simulink model "chap05"  (R2021a)
settings: Solver=FixedStepDiscrete  StartTime=0.0  StopTime=inf  FixedStep=0.001  RelTol=1e-3
undefined symbols (not defined in the file): DiscIntNeverNeededParam, Header, Pose, X, Y, Z
libraries: robotlib x31
(part 9 of 9)

== matlab function chap05/Subsystem16/Subsystem3/Subsystem9/Subsystem/MATLAB Function ==
  data: u1 input; y output; u2 input
function y = fcn(u1,u2)


if (u1==u2)
    y = 0;
else
    y = 1;
end

== matlab function chap05/Subsystem16/Subsystem3/Subsystem3/MATLAB Function ==
  data: u input; y output
function y = fcn(u)

y = u;

if y==0
    y=10e-15;
end

== matlab function chap05/Subsystem16/Subsystem3/Subsystem3/MATLAB Function1 ==
  data: u input; y output
function y = fcn(u)

y = u;

if y==0
    y=10e-15;
end

== matlab function chap05/Subsystem16/Subsystem3/Subsystem3/MATLAB Function2 ==
  data: u input; y output
function y = fcn(u)

y = u;

if y==0
    y=10e-15;
end

== matlab function chap05/Subsystem16/Subsystem3/Subsystem3/Subsystem/MATLAB Function ==
  data: u input; y output
function y = fcn(u)

y = norm(u);

== matlab function chap05/Subsystem16/Subsystem3/Subsystem8/MATLAB Function1 ==
  data: u input; y output
function y = fcn(u)

y = norm(u);

== matlab function chap05/Subsystem16/Subsystem3/Subsystem3/Subsystem1/MATLAB Function ==
  data: u input; y output
function y = fcn(u)

y = norm(u)^(1/2);

== matlab function chap05/Subsystem16/Subsystem5/Subsystem11/Subsystem/MATLAB Function ==
  data: u1 input; y output; u2 input
function y = fcn(u1,u2)


if (u1==u2)
    y = 0;
else
    y = 1;
end

== matlab function chap05/Subsystem16/Subsystem5/Subsystem3/MATLAB Function ==
  data: u input; y output
function y = fcn(u)

y = u;

if y==0
    y=10e-15;
end

== matlab function chap05/Subsystem16/Subsystem5/Subsystem3/MATLAB Function1 ==
  data: u input; y output
function y = fcn(u)

y = u;

if y==0
    y=10e-15;
end

== matlab function chap05/Subsystem16/Subsystem5/Subsystem10/MATLAB Function ==
  data: u input; utk input; nrom output
function nrom = fcn(u,utk)

e = utk-u;
nrom = norm(e);

== matlab function chap05/Subsystem16/Subsystem5/Subsystem3/MATLAB Function2 ==
  data: u input; y output
function y = fcn(u)

y = u;

if y==0
    y=10e-15;
end

== matlab function chap05/Subsystem16/Subsystem5/Subsystem3/Subsystem/MATLAB Function ==
  data: u input; y output
function y = fcn(u)

y = norm(u);

== matlab function chap05/Subsystem16/Subsystem5/Subsystem3/Subsystem1/MATLAB Function ==
  data: u input; y output
function y = fcn(u)

y = norm(u)^(1/2);

== matlab function chap05/Subsystem16/Subsystem5/Subsystem4/Subsystem/MATLAB Function ==
  data: u1 input; y output; u2 input
function y = fcn(u1,u2)


if (u1==u2)
    y = 0;
else
    y = 1;
end

== matlab function chap05/Subsystem16/Subsystem5/Subsystem9/Subsystem/MATLAB Function ==
  data: u1 input; y output; u2 input
function y = fcn(u1,u2)


if (u1==u2)
    y = 0;
else
    y = 1;
end

== matlab function chap05/Subsystem16/Subsystem5/Subsystem7/MATLAB Function ==
  data: u input; y output
function y = fcn(u)

y = norm(u);

== matlab function chap05/Subsystem16/Subsystem6/Subsystem4/Subsystem/MATLAB Function ==
  data: u1 input; y output; u2 input
function y = fcn(u1,u2)


if (u1==u2)
    y = 0;
else
    y = 1;
end

== matlab function chap05/Subsystem16/Subsystem6/Subsystem5/Subsystem/MATLAB Function ==
  data: u1 input; y output; u2 input
function y = fcn(u1,u2)


if (u1==u2)
    y = 0;
else
    y = 1;
end

== matlab function chap05/Subsystem16/Subsystem6/Subsystem7/Subsystem/MATLAB Function ==
  data: u1 input; y output; u2 input
function y = fcn(u1,u2)


if (u1==u2)
    y = 0;
else
    y = 1;
end

== matlab function chap05/Subsystem16/Subsystem1/Subsystem11/Subsystem/MATLAB Function ==
  data: u1 input; y output; u2 input
function y = fcn(u1,u2)


if (u1==u2)
    y = 0;
else
    y = 1;
end

== matlab function chap05/Subsystem16/Subsystem1/Subsystem5/Subsystem/MATLAB Function ==
  data: u1 input; y output; u2 input
function y = fcn(u1,u2)


if (u1==u2)
    y = 0;
else
    y = 1;
end

== matlab function chap05/Subsystem16/Subsystem1/Subsystem9/Subsystem/MATLAB Function ==
  data: u1 input; y output; u2 input
function y = fcn(u1,u2)


if (u1==u2)
    y = 0;
else
    y = 1;
end

== matlab function chap05/Subsystem16/Subsystem12/MATLAB Function ==
  data: u input; y output
function y = fcn(u)

y = norm(u);

== matlab function chap05/Subsystem16/Subsystem12/MATLAB Function2 ==
  data: u input; y output
function y = fcn(u)

y = norm(u);

== matlab function chap05/Subsystem16/Subsystem12/MATLAB Function3 ==
  data: u input; y output
function y = fcn(u)

y = norm(u);

== matlab function chap05/Subsystem16/Subsystem5/Subsystem7/MATLAB Function1 ==
  data: u input; y output
function y = fcn(u)

y = norm(u);

== matlab function chap05/Subsystem16/Subsystem14/MATLAB Function ==
  data: u input; y output
function y = fcn(u)

y = norm(u);

== matlab function chap05/Subsystem16/Subsystem14/MATLAB Function2 ==
  data: u input; y output
function y = fcn(u)

y = norm(u);

== matlab function chap05/Subsystem16/Subsystem14/MATLAB Function3 ==
  data: u input; y output
function y = fcn(u)

y = norm(u);

== matlab function chap05/Subsystem16/Subsystem15/MATLAB Function ==
  data: u input; y output
function y = fcn(u)

y = norm(u);

== matlab function chap05/Subsystem16/Subsystem15/MATLAB Function2 ==
  data: u input; y output
function y = fcn(u)

y = norm(u);

== matlab function chap05/Subsystem16/Subsystem15/MATLAB Function3 ==
  data: u input; y output
function y = fcn(u)

y = norm(u);

== matlab function chap05/Subsystem16/Subsystem16/MATLAB Function ==
  data: u input; y output
function y = fcn(u)

y = norm(u);

== matlab function chap05/Subsystem16/Subsystem16/MATLAB Function2 ==
  data: u input; y output
function y = fcn(u)

y = norm(u);

== matlab function chap05/Subsystem16/Subsystem16/MATLAB Function3 ==
  data: u input; y output
function y = fcn(u)

y = norm(u);

== matlab function chap05/Subsystem16/Subsystem17/MATLAB Function ==
  data: u input; y output
function y = fcn(u)

y = norm(u);

== matlab function chap05/Subsystem16/Subsystem2/Subsystem8/MATLAB Function ==
  data: u input; y output
function y = fcn(u)

y = norm(u);

== matlab function chap05/Subsystem16/Subsystem17/MATLAB Function2 ==
  data: u input; y output
function y = fcn(u)

y = norm(u);

== matlab function chap05/Subsystem16/Subsystem17/MATLAB Function3 ==
  data: u input; y output
function y = fcn(u)

y = norm(u);

== matlab function chap05/Subsystem16/Subsystem8/MATLAB Function ==
  data: u input; y output
function y = fcn(u)

y = norm(u);

== matlab function chap05/Subsystem16/Subsystem8/MATLAB Function2 ==
  data: u input; y output
function y = fcn(u)

y = norm(u);

== matlab function chap05/Subsystem16/Subsystem8/MATLAB Function3 ==
  data: u input; y output
function y = fcn(u)

y = norm(u);

== matlab function chap05/Subsystem16/Subsystem2/Subsystem8/MATLAB Function1 ==
  data: u input; y output
function y = fcn(u)

y = norm(u);

== matlab function chap05/Subsystem16/Subsystem/Subsystem8/MATLAB Function ==
  data: u input; y output
function y = fcn(u)

y = norm(u);

== matlab function chap05/Subsystem16/Subsystem/Subsystem8/MATLAB Function1 ==
  data: u input; y output
function y = fcn(u)

y = norm(u);

== matlab function chap05/Subsystem16/Subsystem1/Subsystem8/MATLAB Function1 ==
  data: u input; y output
function y = fcn(u)

y = norm(u);

== matlab function chap05/Subsystem16/Subsystem2/Subsystem3/Subsystem2/MATLAB Function ==
  data: u input; y output
function y = fcn(u)

y = norm(u);
